simulink model "Three_phase_bridge"  (R2023b)
settings: Solver=FixedStepAuto  StartTime=0.0  StopTime=0.05  FixedStep=1e-6  RelTol=1e-3
libraries: spsDiodeLib x6, spsACVoltageSourceLib x3, spsCurrentMeasurementLib x2, spsVoltageMeasurementLib x2, spsControlledCurrentSourceLib x1, sps_lib x1
settings Model: Creator=N  LastModifiedBy=Ngsanchong
settings OptimizationCC: ReuseModelBlockBuffer=off

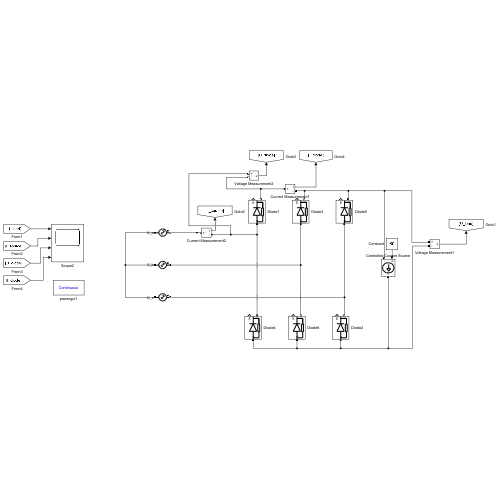
[thumbnail: Simulink's stored preview of the top-level diagram]
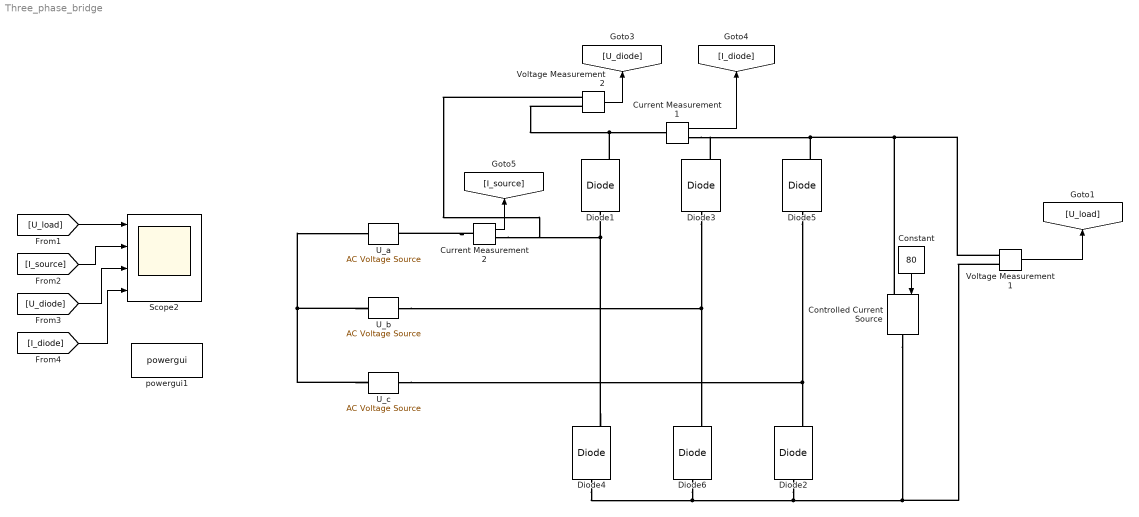
== system Three_phase_bridge ==
  Constant : Constant  Value=80
  Controlled Current Source : spsControlledCurrentSourceLib/Controlled Current Source  Initialize=on  Source_Type=DC  Amplitude=80  Phase=0  Frequency=0  Measurements=None
  Current Measurement1 : spsCurrentMeasurementLib/Current Measurement  PhasorSimulation=off  OutputType=Complex  PSBequivalent=0
  Current Measurement2 : spsCurrentMeasurementLib/Current Measurement  PhasorSimulation=off  OutputType=Complex  PSBequivalent=0
  Diode{1..6} (6 alike) : spsDiodeLib/Diode  Ron=0.001  Lon=0  Vf=0.8  IC=0  UseSnubber=0  Rs=5e5  Cs=250e-9  Measurements=on
  Scope2 : Scope  NumInputPorts=4
  U_a : spsACVoltageSourceLib/AC Voltage Source  Amplitude=68.4*sqrt(2)  Phase=0  Frequency=50  SampleTime=0  Measurements=None  BusType=swing  Pref=10e3  Qref=0  Qmin=-inf  Qmax=+inf
  U_b : spsACVoltageSourceLib/AC Voltage Source  Amplitude=68.4*sqrt(2)  Phase=-120  Frequency=50  SampleTime=0  Measurements=None  BusType=swing  Pref=10e3  Qref=0  Qmin=-inf  Qmax=+inf
  U_c : spsACVoltageSourceLib/AC Voltage Source  Amplitude=68.4*sqrt(2)  Phase=120  Frequency=50  SampleTime=0  Measurements=None  BusType=swing  Pref=10e3  Qref=0  Qmin=-inf  Qmax=+inf
  Voltage Measurement1 : spsVoltageMeasurementLib/Voltage Measurement  PhasorSimulation=off  OutputType=Complex  PSBequivalent=0
  Voltage Measurement2 : spsVoltageMeasurementLib/Voltage Measurement  PhasorSimulation=off  OutputType=Complex  PSBequivalent=0
  powergui1 : sps_lib/powergui  Priority=1  SimulationMode=Continuous  SampleTime=50e-6  frequency=60  Iterations=50  frequencyindice=50  Pbase=100e6  ErrMax=1e-4  UnitsV=kV  UnitsW=MW  buscounter=0  FunctionMessages=off  echomessages=off  EnableUseOfTLC=off  CurrentSourceSwitches=off  DisableSnubberDevices=off  DisableRonSwitches=off  DisableVfSwitches=off  DisplayEquations=off  AutomaticDiscreteSolvers=off  SolverType=Tustin/Backward Euler (TBE)  Interpol=off  ExternalGateDelay=off  methode=off  Ts=100  x0status=blocks  SPID=on  SwTol=0  HookPort=off  NonlinearTolerance=1e-4  nMaxIteration=100  ContinueOnMaxIteration=off  RestoreLinks=warning  ResistiveCurrentMeasurement=off  Frange=[0:2:500]  Ylog=off  Xlog=on  ShowGrid=off  save=off  variable=ZData  structure=0  ZoomFFT=off  StartTime=0.0  cycles=1  DisplayStyle=1  fundamental=60  FreqAxis=off  MaxFrequency=1000  frequencyindicesteady=1  RmsSteady=1  display=off
  wires:
  Voltage Measurement1/1 -> [U_load]
  Current Measurement2/1 -> [I_source]
  Constant/1 -> Controlled Current Source/1
  [I_source] -> Scope2/2
  [U_diode] -> Scope2/3
  [U_load] -> Scope2/1
  [I_diode] -> Scope2/4
  Voltage Measurement2/1 -> [U_diode]
  Current Measurement1/1 -> [I_diode]
  connections:
  Diode4/RConn1 -- Voltage Measurement2/LConn1 -- Current Measurement2/RConn1 -- Diode1/LConn1
  Controlled Current Source/LConn1 -- Voltage Measurement1/LConn1 -- Current Measurement1/RConn1 -- Diode3/RConn1 -- Diode5/RConn1
  Diode3/LConn1 -- U_b/RConn1 -- Diode6/RConn1
  Diode4/LConn1 -- Controlled Current Source/RConn1 -- Voltage Measurement1/LConn2 -- Diode2/LConn1 -- Diode6/LConn1
  Current Measurement2/LConn1 -- U_a/RConn1
  U_b/LConn1 -- U_c/LConn1 -- U_a/LConn1
  Diode5/LConn1 -- U_c/RConn1 -- Diode2/RConn1
  Diode1/RConn1 -- Voltage Measurement2/LConn2 -- Current Measurement1/LConn1
